simulink model "PartitionedController"  (R2021a)
settings: Solver=VariableStepAuto  StartTime=0.0  StopTime=10.0  RelTol=1e-3
undefined symbols (not defined in the file): Kp, Kv
settings Model: Creator=spencercook  LastModifiedBy=pahul
settings SolverCC: AlgebraicLoopSolver=TrustRegion
settings DebuggingCC: SFMachineParentedDataDiag=warning

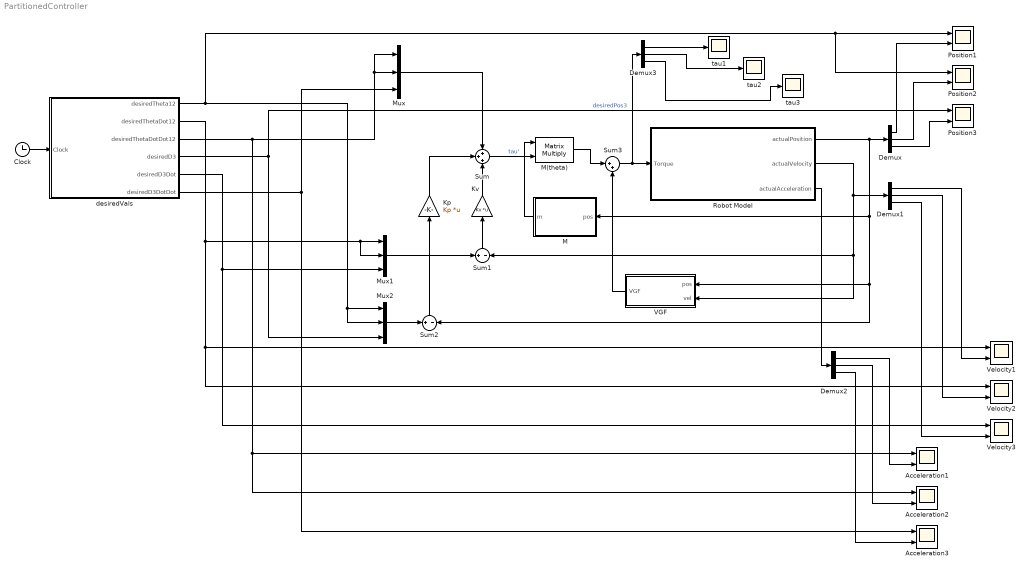
== system PartitionedController ==
  Acceleration1 : Scope  NumInputPorts=2
  Acceleration2 : Scope  NumInputPorts=2
  Acceleration3 : Scope  NumInputPorts=2
  Clock : Clock
  Demux{,1..3} (4 alike) : Demux  Outputs=3
  Kp : Gain  Gain=Kp  Multiplication=Matrix(K*u)
  Kv : Gain  Gain=Kv  Multiplication=Matrix(K*u)
  M : MATLAB Function  TreatAsAtomicUnit=on
  M(theta) : Product  Multiplication=Matrix(*)
  Mux : Mux  Inputs=3
  Mux1 : Mux  Inputs=3
  Mux2 : Mux  Inputs=3
  Position1 : Scope  NumInputPorts=2
  Position2 : Scope  NumInputPorts=2
  Position3 : Scope  NumInputPorts=2
  Robot Model : Subsystem
  Sum : Sum  Inputs=+++
  Sum1 : Sum  Inputs=+|-
  Sum2 : Sum  Inputs=+|-
  Sum3 : Sum  Inputs=|++
  VGF : MATLAB Function  TreatAsAtomicUnit=on
  Velocity1 : Scope  NumInputPorts=2
  Velocity2 : Scope  NumInputPorts=2
  Velocity3 : Scope  NumInputPorts=2
  desiredVals : Subsystem
  tau1 : Scope
  tau2 : Scope
  tau3 : Scope
  wires:
  Kp/1 -> Sum/2
  Kv/1 -> Sum/3
  Sum1/1 -> Kv/1
  Sum2/1 -> Kp/1
  M(theta)/1 -> Sum3/1
  Mux2/1 -> Sum2/1
  VGF/1(VGF) -> Sum3/2
  Mux/1 -> Sum/1
  Mux1/1 -> Sum1/1
  Robot Model/1(actualPosition) -> Demux/1, Sum2/2, VGF/1(pos), M/1(pos)
  Sum3/1 -> Robot Model/1(Torque), Demux3/1
  Robot Model/2(actualVelocity) -> VGF/2(vel), Sum1/2, Demux1/1
  Clock/1 -> desiredVals/1(Clock)
  desiredVals/3(desiredThetaDotDot12) -> Acceleration2/1, Acceleration1/1, Mux/1, Mux/2
  desiredVals/6(desiredD3DotDot) -> Acceleration3/1, Mux/3
  desiredVals/2(desiredThetaDot12) -> Velocity2/1, Velocity1/1, Mux1/2, Mux1/1
  desiredVals/5(desiredD3Dot) -> Velocity3/1, Mux1/3
  desiredVals/1(desiredTheta12) -> Position1/1, Position2/1, Mux2/2, Mux2/1
  desiredVals/4(desiredD3) -> Mux2/3, Position3/1  "desiredPos3"
  Sum/1 -> M(theta)/2  "tau'"
  M/1(m) -> M(theta)/1
  Demux/1 -> Position1/2
  Demux/2 -> Position2/2
  Demux/3 -> Position3/2
  Demux1/1 -> Velocity1/2
  Demux1/2 -> Velocity2/2
  Demux1/3 -> Velocity3/2
  Robot Model/3(actualAcceleration) -> Demux2/1
  Demux2/1 -> Acceleration1/2
  Demux2/2 -> Acceleration2/2
  Demux2/3 -> Acceleration3/2
  Demux3/1 -> tau1/1
  Demux3/2 -> tau2/1
  Demux3/3 -> tau3/1

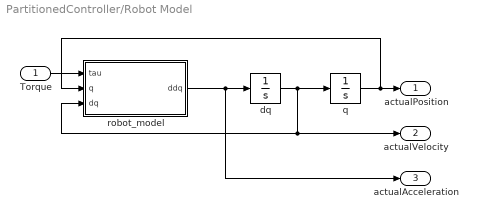
== system PartitionedController/Robot Model ==
  Torque : Inport
  dq : Integrator  InitialCondition=[0 0 -1]
  q : Integrator  InitialCondition=[-pi/4 -pi/4 0.4]
  robot_model : MATLAB Function  TreatAsAtomicUnit=on
  actualPosition : Outport
  actualVelocity : Outport  Port=2
  actualAcceleration : Outport  Port=3
  wires:
  Torque/1 -> robot_model/1(tau)
  q/1 -> robot_model/2(q), actualPosition/1
  robot_model/1(ddq) -> actualAcceleration/1, dq/1
  dq/1 -> q/1, actualVelocity/1, robot_model/3(dq)

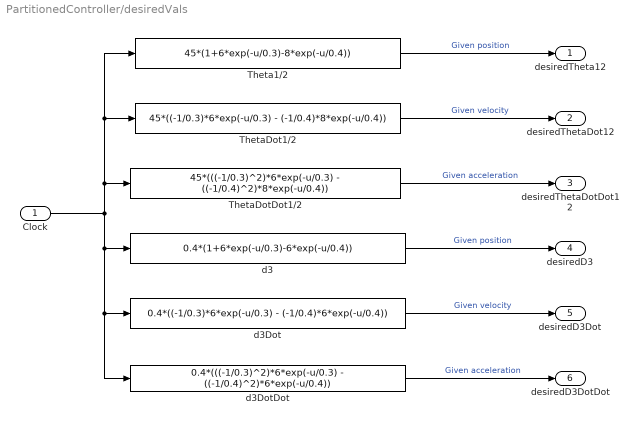
== system PartitionedController/desiredVals ==
  Clock : Inport
  Theta1/2 : Fcn  Expr=45*(1+6*exp(-u/0.3)-8*exp(-u/0.4))
  ThetaDot1/2 : Fcn  Expr=45*((-1/0.3)*6*exp(-u/0.3) - (-1/0.4)*8*exp(-u/0.4))
  ThetaDotDot1/2 : Fcn  Expr=45*(((-1/0.3)^2)*6*exp(-u/0.3) - ((-1/0.4)^2)*8*exp(-u/0.4))
  d3 : Fcn  Expr=0.4*(1+6*exp(-u/0.3)-6*exp(-u/0.4))
  d3Dot : Fcn  Expr=0.4*((-1/0.3)*6*exp(-u/0.3) - (-1/0.4)*6*exp(-u/0.4))
  d3DotDot : Fcn  Expr=0.4*(((-1/0.3)^2)*6*exp(-u/0.3) - ((-1/0.4)^2)*6*exp(-u/0.4))
  desiredTheta12 : Outport
  desiredThetaDot12 : Outport  Port=2
  desiredThetaDotDot12 : Outport  Port=3
  desiredD3 : Outport  Port=4
  desiredD3Dot : Outport  Port=5
  desiredD3DotDot : Outport  Port=6
  wires:
  Clock/1 -> Theta1/2/1, ThetaDot1/2/1, ThetaDotDot1/2/1, d3DotDot/1, d3Dot/1, d3/1
  ThetaDotDot1/2/1 -> desiredThetaDotDot12/1  "Given acceleration"
  ThetaDot1/2/1 -> desiredThetaDot12/1  "Given velocity"
  Theta1/2/1 -> desiredTheta12/1  "Given position"
  d3/1 -> desiredD3/1  "Given position"
  d3Dot/1 -> desiredD3Dot/1  "Given velocity"
  d3DotDot/1 -> desiredD3DotDot/1  "Given acceleration"

== matlab function PartitionedController/Robot Model/robot_model ==
  data: tau input; ddq output; q input; dq input
function ddq = robot_model(tau,q,dq)
ddq=zeros(3,1);
th1=q(1); dth1=dq(1);
th2=q(2); dth2=dq(2);
f=q(3); df=dq(3);
m1=0.08+4*f^2*(sin(th2))^2;
m2=-0.4*f*cos(th2);
m3=-0.2*sin(th2);
m4=4*f^2;
m5=0;
m6=2;

invM = inv([m1 m2 m3; m2 m4 m5; m3 m5 m6]);
size(tau)

V=[0.4*dth2^2*f*sin(th2)-0.4*df*dth2*cos(th2)+8*dth1*dth2*f^2*cos(th2)*sin(th2)+4*df*dth1*f*(sin(th2))^2;...
    -4*dth1^2*f^2*cos(th2)*sin(th2)+4*df*dth2*f;...
	-2*dth1^2*f*(sin(th2))^2-2*dth2^2*f];

G=[0; -4*f*sin(th2)*9.8; 2*cos(th2)*9.8];

ddq = invM*(tau-V-G);

== matlab function PartitionedController/M ==
  data: pos input; m output
function m = interiaMatrix(pos)

theta1 = pos(1); %theta1
theta2 = pos(2); %theta2
d3 = pos(3); %d3

% Calculate m
m1=0.08+4*d3^2*(sin(theta2))^2;
m2=-0.4*d3*cos(theta2);
m3=-0.2*sin(theta2);
m4=4*d3^2;
m5=0;
m6=2;

m = [m1 m2 m3; m2 m4 m5; m3 m5 m6];

== matlab function PartitionedController/VGF ==
  data: pos input; VGF output; vel input
function VGF = calculateVGF(pos,vel)

theta1 = pos(1); %theta1
theta2 = pos(2); %theta2
d3 = pos(3); %d3
theta1_dot = vel(1); % theta1Dot
theta2_dot = vel(2); % theta2Dot
d3_dot = vel(3); % d3Dot

% Calculate V
V=[0.4*theta2_dot^2*d3*sin(theta2)-0.4*d3_dot*theta2_dot*cos(theta2)+8*theta1_dot*theta2_dot*d3^2*cos(theta2)*sin(theta2)+4*d3_dot*theta1_dot*d3*(sin(theta2))^2;...
    -4*theta1_dot^2*d3^2*cos(theta2)*sin(theta2)+4*d3_dot*theta2_dot*d3;...
	-2*theta1_dot^2*d3*(sin(theta2))^2-2*theta2_dot^2*d3];

% Calculate G
G=[0; -4*d3*sin(theta2)*9.8; 2*cos(theta2)*9.8];

VGF = V + G;
